simulink model "Simscape_crane_software_model_SingleContr_R2016b"  (R2016b)
settings: Solver=ode15s  StartTime=0.0  StopTime=180  RelTol=1e-3  EnableMultiTasking=on
values from neighbouring files (symbols this model uses):
  DTraj = 0.3    [RunModel.m]
  ITraj = 0.3    [RunModel.m]
  m = 0.47    [SSmodelParams.mat]
  MR = 1.71    [SSmodelParams.mat]
  PTraj = 3.0    (= 3)    [RunModel.m]
  TxBreak = 0    [setup.m]
  TxCoulomb = 2.5    [setup.m]
  TxVisc = 49.1750    (= 49.175)    [setup.m]
  TyBreak = 0    [setup.m]
  TyCoulomb = 1.8    [setup.m]
  waypoints = vertcat(waypoints, path_to_waypoints(min_path,0))    [path_planning.m]    (also in path_to_waypoints.m = [])
  xZero = 0    [setup.m]
  yZero = 0    [setup.m]
undefined symbols (not defined in the file or in its folder): TzBreak, TzCoulomb, X, xRange, Y, yRange, Z, zRange, zZero
undefined symbols (not defined in the file): M, TorqueMultX, TorqueMultY, TorqueMultZ, TxTrans, TyTrans, TyVisc, TzTrans, TzVisc
libraries: sm_lib x146, fl_lib x62, nesl_utility x24, elec_lib x9, simulink x8, sm_double_wishbone_suspension_lib x4, aerolibtransform2 x1
(part 1 of 14)
settings Model: Creator=jsustare  LastModifiedBy=mc1713
settings SolverCC: MaxConsecutiveMinStep=10
settings DataIOCC: SaveFormat=StructureWithTime
settings OptimizationCC: LifeSpan=inf
settings DebuggingCC: AllowSymbolicDim=off  SFUnexpectedBacktrackingDiag=warning  SFNoUnconditionalDefaultTransitionDiag=warning  SFExecutionAtInitializationDiag=none
settings ModelReferenceCC: PropagateSignalLabelsOutOfModel=off
settings GRTTargetCC: TargetLangStandard=C89/C90 (ANSI)
settings ConfigComp: CovMetricSettings=dw  CovHtmlReporting=on  CovSaveCumulativeToWorkspaceVar=on  CovSaveSingleToWorkspaceVar=on  CovExternalEMLEnable=off
settings SimscapeCC: SimscapeLogType=all
settings ConfigurationSet: Description=SimMechanics 2G

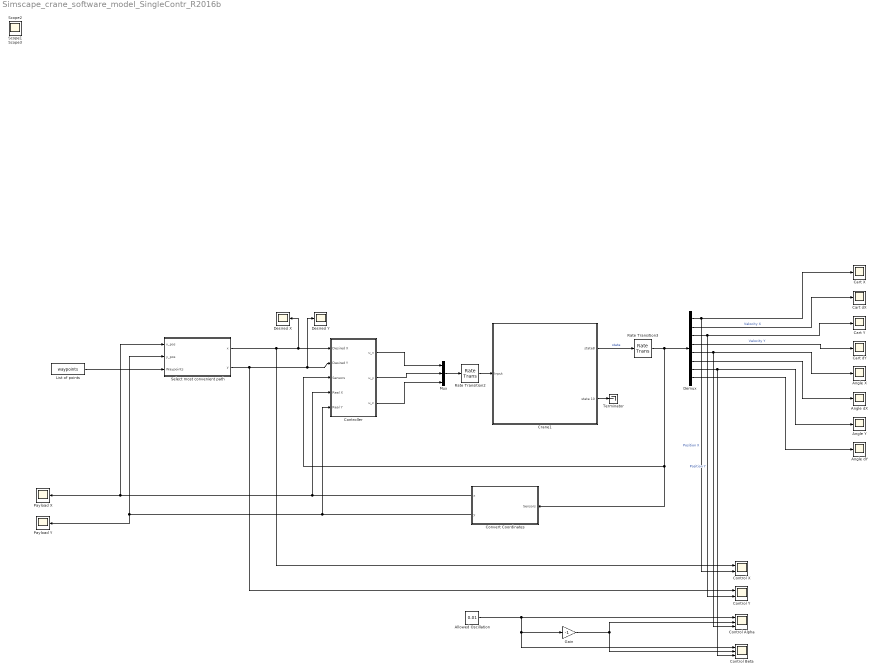
== system Simscape_crane_software_model_SingleContr_R2016b ==
  Allowed Oscillation : Constant  Value=0.01
  Angle X : Scope
  Angle Y : Scope
  Angle dX : Scope
  Angle dY : Scope
  Cart X : Scope
  Cart Y : Scope
  Cart dX : Scope
  Cart dY : Scope
  Control Alpha : Scope  NumInputPorts=3
  Control Beta : Scope  NumInputPorts=3
  Control X : Scope  NumInputPorts=2
  Control Y : Scope  NumInputPorts=2
  Controller : Subsystem
  Convert Coordinates : MATLAB Function  TreatAsAtomicUnit=on
  Crane1 : Subsystem  mask{penduMass=m, cartMass=M, MR=MR, xRange=xRange, yRange=yRange, zRange=zRange, xZero=xZero, yZero=yZero, zZero=zZero, TxBreak=TxBreak, TxCoulomb=TxCoulomb, TxVisc=TxVisc, TxTrans=TxTrans, TyBreak=TyBreak, TyCoulomb=TyCoulomb, TyVisc=TyVisc, TyTrans=TyTrans, TzBreak=TzBreak, TzCoulomb=TzCoulomb, TzVisc=TzVisc, TzTrans=TzTrans, Ux=TorqueMultX, Uy=TorqueMultY, Uz=TorqueMultZ}
      mask prompts: penduMass "Pendulum Mass (Kg)"; cartMass "Mass of the cart (Kg)"; MR "Mass of the rail (Kg)"; TxBreak "BreakAwayFriction"; TxCoulomb "Coulomb Friction"; TxVisc "Viscous friction"; TxTrans "Transition coeff"; TyBreak "BreakAwayFriction"; TyCoulomb "Coulomb Friction"; TyVisc "Viscous friction"; TyTrans "Transition coeff"; TzBreak "BreakAwayFriction"; TzCoulomb "Coulomb Friction"; TzVisc "Viscous friction"; TzTrans "Transition coeff"; Ux "Rail motor multiplier (X)"; Uy "Cart motor multiplier (Y)"; Uz "String motor multiplier (Z)"
      mask init:
      | %mass lowSat
      | penduMass=max(penduMass,1e-3);
      | cartMass=max(cartMass,1e-3);
      | MR=max(MR,1e-3);
      | 
      | %zeros saturated
      | xZero=max(xZero,xRange(1));
      | xZero=min(xZero,xRange(2));
      | 
      | yZero=max(yZero,yRange(1));
      | yZero=min(yZero,yRange(2));
      | 
      | zZero=max(zZero,zRange(1));
      | zZero=min(zZero,zRange(2));
      mask DialogControl DescGroupVar Prompt: 3D Crane Simscape model
      mask Display:
